simulink model "hopper_3dof_cascade_No_wind - Copy"  (R2025a)
settings: Solver=VariableStepAuto  StartTime=0.0  StopTime=60  MaxStep=.005  RelTol=1e-3
values from neighbouring files (symbols this model uses):
  AVI = size_avionics(IN)    [main.m]
  bp = data(:,1)    [load_lookup.m]
  ENGINE = size_engine(IN)    [main.m]
  IN =     [hopper_sizing_output.mat]    (also in main.m = mission_inputs())
  OUT =     [hopper_sizing_output.mat]    (also in main.m = Outputs(IN, VEH, TANKS, STRUCT))
  TANKS = size_tanks(IN)    [main.m]
undefined symbols (not defined in the file or in its folder): tbl1, tbl2
libraries: slpidlib x5, simulink x4, SignalEditorBlockLib x1, cstblocks x1, dspsrcs4 x1
settings Model: Creator=Espin  LastModifiedBy=Espin
settings DebuggingCC: AlgebraicLoopMsg=none

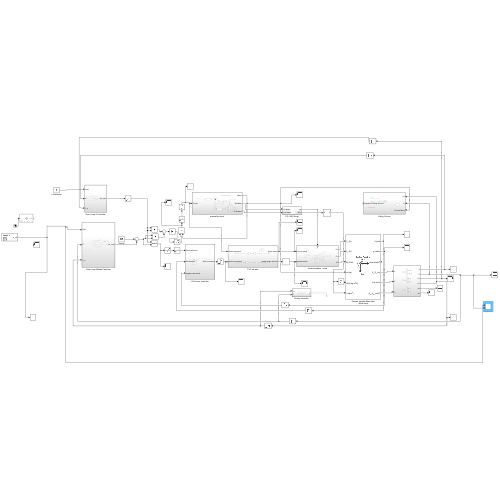
[thumbnail: Simulink's stored preview of the top-level diagram]
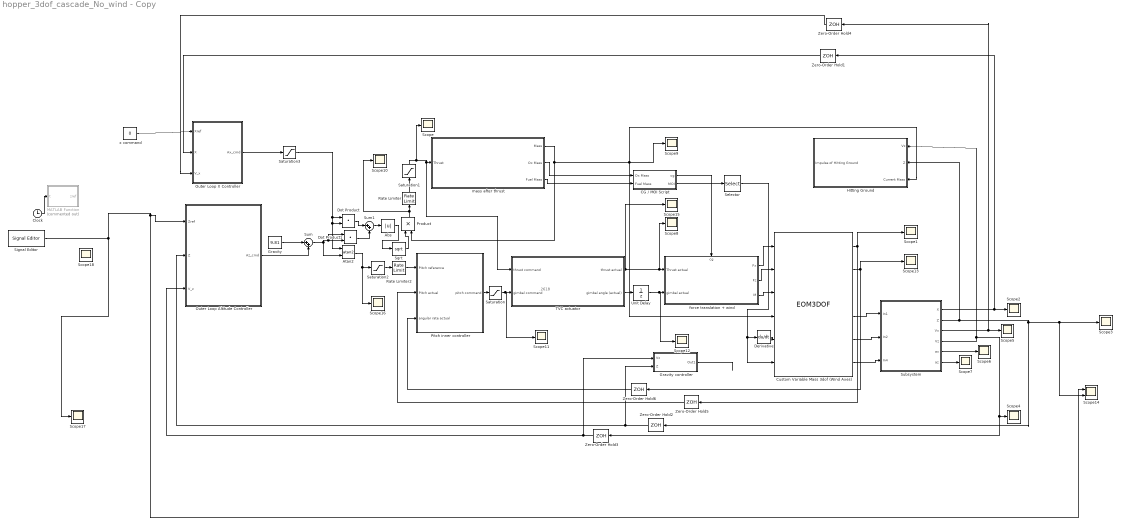
== system hopper_3dof_cascade_No_wind - Copy ==
  note: .2618
  Abs : Abs  SaturateOnIntegerOverflow=off
  Atan2 : Trigonometry  Operator=atan2
  CG / MOI Script : Subsystem
  Clock : Clock
  Custom Variable Mass 3dof (Wind Axes) : EOM3DOF  mtype=Custom Variable  v_ini=0
  Derivative : Derivative
  Dot Product : DotProduct  OutDataTypeStr=Inherit: Inherit via internal rule
  Dot Product1 : DotProduct  OutDataTypeStr=Inherit: Inherit via internal rule
  Gravity : Constant  Value=9.81
  Gravity controller : Subsystem
  Hitting Ground : Subsystem
  MATLAB Function : MATLAB Function  Commented=on  TreatAsAtomicUnit=on
  Outer Loop Altitude Controller : Subsystem
  Outer Loop X Controller : Subsystem
  Pitch inner controller : Subsystem
  Product : Product
  Rate Limiter : RateLimiter  RisingSlewLimit=800  FallingSlewLimit=-800  SampleTimeMode=inherited
  Rate Limiter2 : RateLimiter  RisingSlewLimit=.2618  FallingSlewLimit=-.2618  SampleTimeMode=inherited
  Saturation : Saturate  UpperLimit=.25  LowerLimit=-.25
  Saturation1 : Saturate  UpperLimit=2400  LowerLimit=890  ZeroCross=off
  Saturation2 : Saturate  UpperLimit=.1  LowerLimit=-.1
  Saturation3 : Saturate  UpperLimit=.8  LowerLimit=-.8
  Scope{,1..13,15..18} (18 alike) : Scope
      Scope settings: ActiveDisplayYMinimum=624.4996725299402  ActiveDisplayYMaximum=2705.46842252994  DataLoggingVariableName=ScopeData17
      Scope1 settings: ActiveDisplayYMinimum=-3.9694175819180568  ActiveDisplayYMaximum=3.8842046224775704  DataLoggingVariableName=ScopeData4
      Scope10 settings: ActiveDisplayYMinimum=-1  ActiveDisplayYMaximum=1  DataLoggingVariableName=ScopeData18
      Scope11 settings: ActiveDisplayYMinimum=-0.486354941657661  ActiveDisplayYMaximum=0.24913214764343761  DataLoggingVariableName=ScopeData19
      Scope12 settings: ActiveDisplayYMinimum=-1.2645796500990321  ActiveDisplayYMaximum=0.59395959390663888  DataLoggingVariableName=ScopeData20
      Scope13 settings: ActiveDisplayYMinimum=0.23771889209507596  ActiveDisplayYMaximum=0.35709262601864444  DataLoggingVariableName=ScopeData21
      Scope15 settings: ActiveDisplayYMinimum=931.27769507113021  ActiveDisplayYMaximum=1211.8430429766809  DataLoggingVariableName=ScopeData25
      Scope16 settings: ActiveDisplayYMinimum=-0.10872394180597797  ActiveDisplayYMaximum=0.024612722486554474  DataLoggingVariableName=ScopeData26
      Scope17 settings: ActiveDisplayYMinimum=-6.2499999999999982  ActiveDisplayYMaximum=56.25  DataLoggingVariableName=ScopeData31
      Scope18 settings: ActiveDisplayYMinimum=-6.2499999999999982  ActiveDisplayYMaximum=56.25  DataLoggingVariableName=ScopeData39
      Scope2 settings: ActiveDisplayYMinimum=-3413.3164906748493  ActiveDisplayYMaximum=7586.6291552550156  DataLoggingVariableName=ScopeData6
      Scope3 settings: ActiveDisplayYMinimum=-1202.9630045130734  ActiveDisplayYMaximum=1936.8327091689698  DataLoggingVariableName=ScopeData7
      Scope4 settings: ActiveDisplayYMinimum=-29.297460678782883  ActiveDisplayYMaximum=38.963570912357639
      Scope5 settings: ActiveDisplayYMinimum=-962.2230612403514  ActiveDisplayYMaximum=1558.6587762750428  DataLoggingVariableName=ScopeData9
      Scope6 settings: ActiveDisplayYMinimum=-962.2230612403514  ActiveDisplayYMaximum=1558.6587762750428  DataLoggingVariableName=ScopeData10
      Scope7 settings: ActiveDisplayYMinimum=-962.2230612403514  ActiveDisplayYMaximum=1558.6587762750428  DataLoggingVariableName=ScopeData11
      Scope8 settings: ActiveDisplayYMinimum=931.27769507113021  ActiveDisplayYMaximum=1211.8430429766809  DataLoggingVariableName=ScopeData12
      Scope9 settings: ActiveDisplayYMinimum=94.915833260187526  ActiveDisplayYMaximum=94.915892608014829  DataLoggingVariableName=ScopeData13
  Scope14 : Scope  NumInputPorts=2
      settings: ActiveDisplayYMinimum=-2.6899782864025186  ActiveDisplayYMaximum=3.1359753018738186  DataLoggingVariableName=ScopeData22
  Selector : Selector  NumberOfDimensions=2  InputPortWidth=1  IndexOptions=Index vector (dialog),Index vector (dialog)  Indices=2,2  OutputSizes=1,1
  Signal Editor : SignalEditorBlockLib/Signal Editor  FileName=trajectory2.mat  ActiveScenario=scenario  ActiveSignal=z_ref  IsBus=off  OutputBusObjectStr=Bus: BusObject  SampleTime=0  ZeroCross=off  OutputAfterFinalValue=Setting to zero  Unit=inherit  PreserveSignalName=on  ApplySigPropsToAllScenarios=on  ApplySigPropsToAllSignals=off  SignalPropertySource=Dialog parameters
  Sqrt : Sqrt
  Subsystem : Subsystem
  Sum : Sum  Inputs=|++
  Sum1 : Sum  Inputs=|++
  TVC actuator : Subsystem
  Unit Delay : UnitDelay  SampleTime=-1  HasFrameUpgradeWarning=on
  Zero-Order Hold{1..6} (6 alike) : ZeroOrderHold  SampleTime=-1
  force translation + wind : Subsystem
      settings: PortSchema="{\"entries\":[{\"content\":{\"sides\":[{\"content\":{\"connectorIds\":[\"In1\",\"In2\"]},\"type\":\"ConnectorPlacement.EquallySpacedRectSide\",\"uuid\":\"479fd6fb-19b9-4dfd-bf6b-42f12e82a54f\"},{\"content\":{\"connectorIds\":[\"Out1\",\"Out2\",\"Out3\"],\"side\":\"RIGHT\"},\"type\":\"ConnectorPlacement.EquallySpacedRectSide\",\"uuid\":\"4df03b8d-1b7e-4664-b5ef-d45791de0677\"},{\"content\":{\"connectorIds\":[\"In3\"],\"side\":\"TOP\"},\"type\":\"ConnectorPlacement.EquallySpacedRectSide\",\"uuid\":\"8e173f4c-8dd7-429b-b7ff-7241e32a3938\"}]},\"type\":\"ConnectorPlacement.EquallySpacedConnector\",\"uuid\":\"4fb4042b-69d2-4473-a071-5f8ab2a018ab\"}],\"packageUris\":[\"http://schema.mathworks.com/mf0/Connector/R2020b\"],\"version\":\"1.0\"}"
  mass after thrust : Subsystem
  x command : Constant  Value=0
  wires:
  Custom Variable Mass 3dof (Wind Axes)/6 -> Subsystem/3(In4)
  Custom Variable Mass 3dof (Wind Axes)/5 -> Subsystem/2(In2)
  Custom Variable Mass 3dof (Wind Axes)/4 -> Subsystem/1(In1)
  Atan2/1 -> Scope16/1, Saturation2/1
  Pitch inner controller/1(pitch command) -> Saturation/1
  Saturation/1 -> Scope11/1, TVC actuator/2(gimbal command)
  Gravity/1 -> Sum/1
  mass after thrust/1(Mass) -> Product/2, Hitting Ground/3(Current Mass), Scope9/1, Custom Variable Mass 3dof (Wind Axes)/4
  Rate Limiter/1 -> Saturation1/1
  Product/1 -> Scope10/1, Rate Limiter/1
  Custom Variable Mass 3dof (Wind Axes)/1 -> Scope1/1, Zero-Order Hold5/1
  Custom Variable Mass 3dof (Wind Axes)/2 -> Scope13/1, Zero-Order Hold6/1
  Subsystem/1(X) -> Zero-Order Hold1/1, Scope2/1
  Subsystem/2(Z) -> Hitting Ground/2(Z), Zero-Order Hold2/1, Scope14/2, Scope3/1
  force translation + wind/1(Fx) -> Custom Variable Mass 3dof (Wind Axes)/1
  force translation + wind/3(M) -> Custom Variable Mass 3dof (Wind Axes)/3
  force translation + wind/2(Fz) -> Custom Variable Mass 3dof (Wind Axes)/2
  Subsystem/4(Vz) -> Hitting Ground/1(Vz), Zero-Order Hold3/1, Scope4/1
  Subsystem/3(Vx) -> Zero-Order Hold4/1, Scope5/1
  Subsystem/5(ax) -> Scope6/1
  Subsystem/6(az) -> Scope7/1
  Signal Editor/1 -> Scope14/1, Outer Loop Altitude Controller/1(Zref), Scope17/1
  Outer Loop Altitude Controller/1(Az_cmd) -> Sum/2
  Sqrt/1 -> Product/1
  x command/1 -> Outer Loop X Controller/1(Xref)
  Sum/1 -> Dot Product1/1, Dot Product1/2, Atan2/2
  Dot Product/1 -> Sum1/1
  Sum1/1 -> Abs/1
  Dot Product1/1 -> Sum1/2
  Abs/1 -> Sqrt/1
  Outer Loop X Controller/1(Ax_cmd) -> Saturation3/1
  Saturation1/1 -> Scope/1, TVC actuator/1(thrust command), mass after thrust/1(Thrust)
  Zero-Order Hold1/1 -> Outer Loop X Controller/2(X)
  Zero-Order Hold4/1 -> Outer Loop X Controller/3(V_x)
  Zero-Order Hold3/1 -> Gravity controller/1(Vz), Outer Loop Altitude Controller/3(V_z)
  Zero-Order Hold2/1 -> Gravity controller/2(Z), Outer Loop Altitude Controller/2(Z)
  Zero-Order Hold5/1 -> Pitch inner controller/2(Pitch actual)
  Zero-Order Hold6/1 -> Pitch inner controller/3(angular rate actual)
  TVC actuator/2(gimbal angle (actual)) -> Unit Delay/1
  Unit Delay/1 -> Scope12/1, force translation + wind/2(gimbal actual)
  TVC actuator/1(thrust actual) -> Scope8/1, force translation + wind/1(Thrust actual), Scope15/1
  Saturation2/1 -> Rate Limiter2/1
  Rate Limiter2/1 -> Pitch inner controller/1(Pitch reference)
  Saturation3/1 -> Dot Product/1, Atan2/1, Dot Product/2
  mass after thrust/2(Ox Mass) -> CG / MOI Script/1(Ox Mass)
  mass after thrust/3(Fuel Mass) -> CG / MOI Script/2(Fuel Mass)
  CG / MOI Script/1(cg) -> force translation + wind/3(cg)
  Derivative/1 -> Custom Variable Mass 3dof (Wind Axes)/5
  CG / MOI Script/2(MOI) -> Selector/1
  Selector/1 -> Custom Variable Mass 3dof (Wind Axes)/6, Derivative/1
  Clock/1 -> MATLAB Function/1(t)
  Gravity controller/1(Out1) -> ?

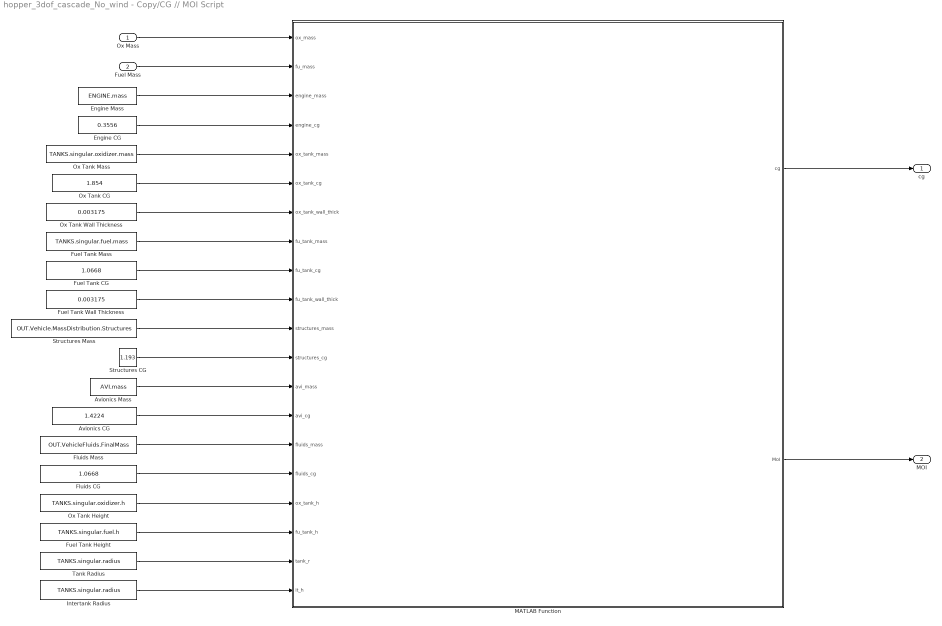
== system hopper_3dof_cascade_No_wind - Copy/CG // MOI Script ==
  Ox Mass : Inport
  Fuel Mass : Inport  Port=2
  Avionics CG : Constant  Value=1.4224
  Avionics Mass : Constant  Value=AVI.mass
  Engine CG : Constant  Value=0.3556
  Engine Mass : Constant  Value=ENGINE.mass
  Fluids CG : Constant  Value=1.0668
  Fluids Mass : Constant  Value=OUT.VehicleFluids.FinalMass
  Fuel Tank CG : Constant  Value=1.0668
  Fuel Tank Height : Constant  Value=TANKS.singular.fuel.h
  Fuel Tank Mass : Constant  Value=TANKS.singular.fuel.mass
  Fuel Tank Wall Thickness : Constant  Value=0.003175
  Intertank Radius : Constant  Value=TANKS.singular.radius
  MATLAB Function : MATLAB Function  TreatAsAtomicUnit=on
  Ox Tank CG : Constant  Value=1.854
  Ox Tank Height : Constant  Value=TANKS.singular.oxidizer.h
  Ox Tank Mass : Constant  Value=TANKS.singular.oxidizer.mass
  Ox Tank Wall Thickness : Constant  Value=0.003175
  Structures CG : Constant  Value=1.193
  Structures Mass : Constant  Value=OUT.Vehicle.MassDistribution.Structures
  Tank Radius : Constant  Value=TANKS.singular.radius
  cg : Outport
  MOI : Outport  Port=2
  wires:
  Ox Mass/1 -> MATLAB Function/1(ox_mass)
  Fuel Mass/1 -> MATLAB Function/2(fu_mass)
  Engine Mass/1 -> MATLAB Function/3(engine_mass)
  Engine CG/1 -> MATLAB Function/4(engine_cg)
  Ox Tank Mass/1 -> MATLAB Function/5(ox_tank_mass)
  Ox Tank CG/1 -> MATLAB Function/6(ox_tank_cg)
  Ox Tank Wall Thickness/1 -> MATLAB Function/7(ox_tank_wall_thick)
  Fuel Tank Mass/1 -> MATLAB Function/8(fu_tank_mass)
  Fuel Tank CG/1 -> MATLAB Function/9(fu_tank_cg)
  Fuel Tank Wall Thickness/1 -> MATLAB Function/10(fu_tank_wall_thick)
  Structures Mass/1 -> MATLAB Function/11(structures_mass)
  Structures CG/1 -> MATLAB Function/12(structures_cg)
  Avionics Mass/1 -> MATLAB Function/13(avi_mass)
  Avionics CG/1 -> MATLAB Function/14(avi_cg)
  Fluids Mass/1 -> MATLAB Function/15(fluids_mass)
  Fluids CG/1 -> MATLAB Function/16(fluids_cg)
  Ox Tank Height/1 -> MATLAB Function/17(ox_tank_h)
  Fuel Tank Height/1 -> MATLAB Function/18(fu_tank_h)
  Tank Radius/1 -> MATLAB Function/19(tank_r)
  Intertank Radius/1 -> MATLAB Function/20(it_h)
  MATLAB Function/2(MoI) -> MOI/1
  MATLAB Function/1(cg) -> cg/1

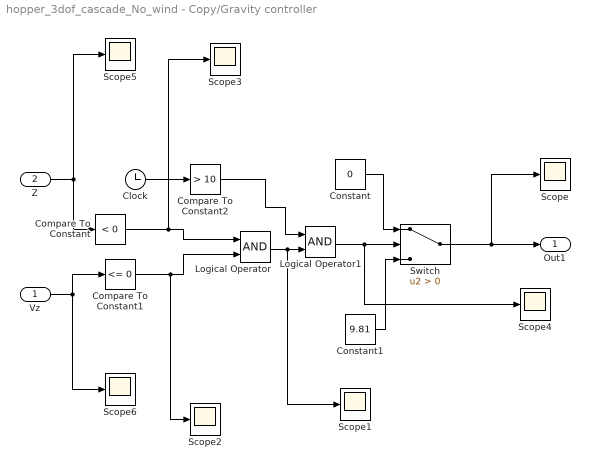
== system hopper_3dof_cascade_No_wind - Copy/Gravity controller ==
  Vz : Inport
  Z : Inport  Port=2
  Clock : Clock
  Compare To Constant : simulink/Logic and Bit Operations/Compare To Constant  relop=<  const=0  OutDataTypeStr=boolean
  Compare To Constant1 : simulink/Logic and Bit Operations/Compare To Constant  relop=<=  const=0  OutDataTypeStr=boolean
  Compare To Constant2 : simulink/Logic and Bit Operations/Compare To Constant  relop=>  const=10  OutDataTypeStr=boolean
  Constant : Constant  Value=0
  Constant1 : Constant  Value=9.81
  Logical Operator : Logic  AllPortsSameDT=off  OutDataTypeStr=boolean
  Logical Operator1 : Logic  AllPortsSameDT=off  OutDataTypeStr=boolean
  Scope{,1..6} (7 alike) : Scope
      Scope settings: ActiveDisplayYMinimum=-0.8627829911971161  ActiveDisplayYMaximum=3.9899046567195673  DataLoggingVariableName=ScopeData32
      Scope1 settings: ActiveDisplayYMinimum=-1  ActiveDisplayYMaximum=1  DataLoggingVariableName=ScopeData33
      Scope2 settings: ActiveDisplayYMinimum=-1  ActiveDisplayYMaximum=1  DataLoggingVariableName=ScopeData34
      Scope3 settings: ActiveDisplayYMinimum=0.16297275299479574  ActiveDisplayYMaximum=1.8744028088981914  DataLoggingVariableName=ScopeData35
      Scope4 settings: ActiveDisplayYMinimum=-1  ActiveDisplayYMaximum=1  DataLoggingVariableName=ScopeData36
      Scope5 settings: ActiveDisplayYMinimum=-1.0594311377245509  ActiveDisplayYMaximum=1.0405688622754492  DataLoggingVariableName=ScopeData37
      Scope6 settings: ActiveDisplayYMinimum=-1.2262499999999998  ActiveDisplayYMaximum=11.03625  DataLoggingVariableName=ScopeData38
  Switch : Switch  Criteria=u2 > Threshold  SaturateOnIntegerOverflow=off  InputSameDT=off
  Out1 : Outport
  wires:
  Vz/1 -> Scope6/1, Compare To Constant1/1
  Z/1 -> Scope5/1, Compare To Constant/1
  Compare To Constant1/1 -> Scope2/1, Logical Operator/2
  Compare To Constant/1 -> Scope3/1, Logical Operator/1
  Clock/1 -> Compare To Constant2/1
  Compare To Constant2/1 -> Logical Operator1/1
  Logical Operator/1 -> Scope1/1, Logical Operator1/2
  Logical Operator1/1 -> Scope4/1, Switch/2
  Constant1/1 -> Switch/3
  Constant/1 -> Switch/1
  Switch/1 -> Scope/1, Out1/1

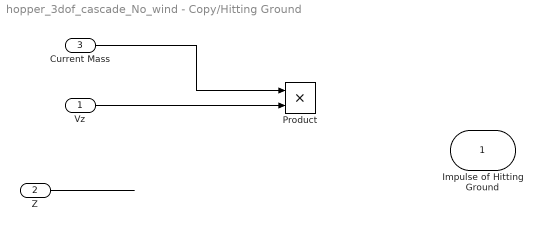
== system hopper_3dof_cascade_No_wind - Copy/Hitting Ground ==
  Vz : Inport
  Z : Inport  Port=2
  Current Mass : Inport  Port=3
  Product : Product
  Impulse of Hitting Ground : Outport
  wires:
  Vz/1 -> Product/2
  Z/1 -> ?
  Current Mass/1 -> Product/1

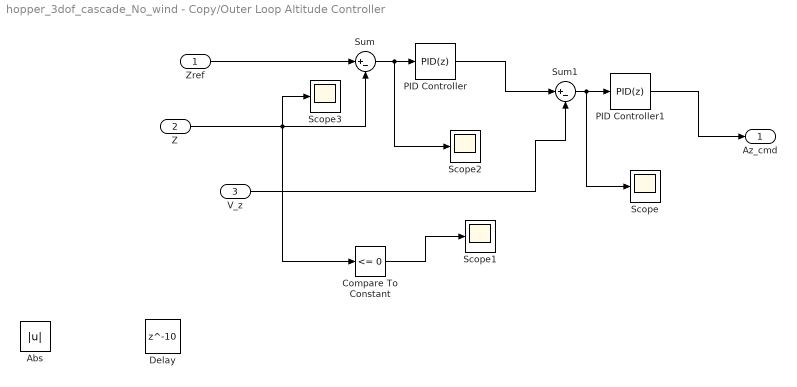
== system hopper_3dof_cascade_No_wind - Copy/Outer Loop Altitude Controller ==
  Zref : Inport
  Z : Inport  Port=2
  V_z : Inport  Port=3
  Abs : Abs  SaturateOnIntegerOverflow=off
  Compare To Constant : simulink/Logic and Bit Operations/Compare To Constant  relop=<=  const=0  OutDataTypeStr=boolean
  Delay : Delay  DelayLength=10  InitialCondition=0
  PID Controller : slpidlib/PID Controller  Controller=PID  Form=Parallel  TimeDomain=Discrete-time  UseExternalTs=off  SampleTime=.02  IntegratorMethod=Forward Euler  FilterMethod=Forward Euler  ControllerParametersSource=internal  P=1  I=0  UseKiTs=off  D=0  UseExternalDerivativeSource=off  N=71.8360137365129  UseFilter=off  TunerSelectOption=Transfer Function Based (PID Tuner App)  InitialConditionSource=internal  InitialConditionForIntegrator=0  InitialConditionForFilter=0  DifferentiatorICPrevScaledInput=0  ExternalReset=none  TrackingMode=off  Kt=1  LimitOutput=off  SatLimitsSource=internal  UpperSaturationLimit=inf  LowerSaturationLimit=-inf  LinearizeAsGain=on  AntiWindupMode=none  Kb=1  LimitIntegrator=off  UpperIntegratorSaturationLimit=inf  LowerIntegratorSaturationLimit=-inf  POutMin=[]  POutMax=[]  IOutMin=[]  IOutMax=[]  DOutMin=[]  DOutMax=[]  NOutMin=[]  NOutMax=[]  SumOutMin=[]  SumOutMax=[]  SaturationOutMin=[]  SaturationOutMax=[]  PParamMin=[]  PParamMax=[]  IParamMin=[]  IParamMax=[]  DParamMin=[]  DParamMax=[]  NParamMin=[]  NParamMax=[]  KbParamMin=[]  KbParamMax=[]  KtParamMin=[]  KtParamMax=[]  KbOutMin=[]  KbOutMax=[]  KtOutMin=[]  KtOutMax=[]  IntegratorOutMin=[]  IntegratorOutMax=[]  FilterOutMin=[]  FilterOutMax=[]  SumI1OutMin=[]  SumI1OutMax=[]  SumI2OutMin=[]  SumI2OutMax=[]  SumI3OutMin=[]  SumI3OutMax=[]  SumI4OutMin=[]  SumI4OutMax=[]  SumDOutMin=[]  SumDOutMax=[]  DifferentiatorOutMin=[]  DifferentiatorOutMax=[]  FilterDiffOutCoefMin=[]  FilterDiffOutCoefMax=[]  ReciprocalOutMin=[]  ReciprocalOutMax=[]  SumDenOutMin=[]  SumDenOutMax=[]  SumNumOutMin=[]  SumNumOutMax=[]  DivideOutMin=[]  DivideOutMax=[]  UdiffTsProdOutMin=[]  UdiffTsProdOutMax=[]  NTsProdOutMin=[]  NTsProdOutMax=[]  UintegralTsProdOutMin=[]  UintegralTsProdOutMax=[]  UngainTsProdOutMin=[]  UngainTsProdOutMax=[]  ClampingZeroOutDataTypeStr=Inherit: Inherit via back propagation  ClampingZeroOutMin=[]  ClampingZeroOutMax=[]  FilterDenConstantOutDataTypeStr=Inherit: Inherit via back propagation  FilterDenConstantOutMin=[]  FilterDenConstantOutMax=[]  PCopyOutDataTypeStr=Inherit: Inherit via back propagation  PCopyOutMin=[]  PCopyOutMax=[]  NCopyOutDataTypeStr=Inherit: Inherit via back propagation  NCopyOutMin=[]  NCopyOutMax=[]  IntegratorContinuousStateAttributes=''  IntegratorStateMustResolveToSignalObject=off  IntegratorRTWStateStorageClass=Auto  FilterContinuousStateAttributes=''  FilterStateMustResolveToSignalObject=off  FilterRTWStateStorageClass=Auto  ParallelPVariant=InternalParameters  IdealPVariant=Disabled  IVariant=InternalParameters  DVariant=InternalParameters  IntegratorVariant=Discrete  SatVariant=Disabled  AWVariant=Passthrough  PCopyVariant=Disabled  TRVariant=Disabled  FdbkBlocksVariant=Forward  IdealPFdbkVariant=Disabled  SatFdbkVariant=Disabled  DerivativeFilterVariant=Differentiator  NVariant=Passthrough  NCopyVariant=Disabled_SignalSpec  FilterICVariant=InternalICsDifferentiator  IntegratorICVariant=InternalICs  ExternalResetVariant=Disabled  TRSumVariant=Passthrough  SumFdbkVariant=Disabled  SumVariant=Sum_PID  TsampFilterVariant=InternalTs  TsampNgainVariant=Passthrough  TsampIntegralVariant=Disabled_SignalSpec  ExternalSaturationOutDataTypeStr=Inherit: Same as second input  DerivativeSourceVariant=ErrorSignal  PreIntVariant=InternalPreInt
  PID Controller1 : slpidlib/PID Controller  Controller=PID  Form=Parallel  TimeDomain=Discrete-time  UseExternalTs=off  SampleTime=.02  IntegratorMethod=Forward Euler  FilterMethod=Forward Euler  ControllerParametersSource=internal  P=-4.85683929346037  I=-2.4299931951401  UseKiTs=off  D=-0.135933719312933  UseExternalDerivativeSource=off  N=71.8360137365129  UseFilter=off  TunerSelectOption=Transfer Function Based (PID Tuner App)  InitialConditionSource=internal  InitialConditionForIntegrator=0  InitialConditionForFilter=0  DifferentiatorICPrevScaledInput=0  ExternalReset=none  TrackingMode=off  Kt=1  LimitOutput=off  SatLimitsSource=internal  UpperSaturationLimit=inf  LowerSaturationLimit=-inf  LinearizeAsGain=on  AntiWindupMode=none  Kb=1  LimitIntegrator=off  UpperIntegratorSaturationLimit=inf  LowerIntegratorSaturationLimit=-inf  POutMin=[]  POutMax=[]  IOutMin=[]  IOutMax=[]  DOutMin=[]  DOutMax=[]  NOutMin=[]  NOutMax=[]  SumOutMin=[]  SumOutMax=[]  SaturationOutMin=[]  SaturationOutMax=[]  PParamMin=[]  PParamMax=[]  IParamMin=[]  IParamMax=[]  DParamMin=[]  DParamMax=[]  NParamMin=[]  NParamMax=[]  KbParamMin=[]  KbParamMax=[]  KtParamMin=[]  KtParamMax=[]  KbOutMin=[]  KbOutMax=[]  KtOutMin=[]  KtOutMax=[]  IntegratorOutMin=[]  IntegratorOutMax=[]  FilterOutMin=[]  FilterOutMax=[]  SumI1OutMin=[]  SumI1OutMax=[]  SumI2OutMin=[]  SumI2OutMax=[]  SumI3OutMin=[]  SumI3OutMax=[]  SumI4OutMin=[]  SumI4OutMax=[]  SumDOutMin=[]  SumDOutMax=[]  DifferentiatorOutMin=[]  DifferentiatorOutMax=[]  FilterDiffOutCoefMin=[]  FilterDiffOutCoefMax=[]  ReciprocalOutMin=[]  ReciprocalOutMax=[]  SumDenOutMin=[]  SumDenOutMax=[]  SumNumOutMin=[]  SumNumOutMax=[]  DivideOutMin=[]  DivideOutMax=[]  UdiffTsProdOutMin=[]  UdiffTsProdOutMax=[]  NTsProdOutMin=[]  NTsProdOutMax=[]  UintegralTsProdOutMin=[]  UintegralTsProdOutMax=[]  UngainTsProdOutMin=[]  UngainTsProdOutMax=[]  ClampingZeroOutDataTypeStr=Inherit: Inherit via back propagation  ClampingZeroOutMin=[]  ClampingZeroOutMax=[]  FilterDenConstantOutDataTypeStr=Inherit: Inherit via back propagation  FilterDenConstantOutMin=[]  FilterDenConstantOutMax=[]  PCopyOutDataTypeStr=Inherit: Inherit via back propagation  PCopyOutMin=[]  PCopyOutMax=[]  NCopyOutDataTypeStr=Inherit: Inherit via back propagation  NCopyOutMin=[]  NCopyOutMax=[]  IntegratorContinuousStateAttributes=''  IntegratorStateMustResolveToSignalObject=off  IntegratorRTWStateStorageClass=Auto  FilterContinuousStateAttributes=''  FilterStateMustResolveToSignalObject=off  FilterRTWStateStorageClass=Auto  ParallelPVariant=InternalParameters  IdealPVariant=Disabled  IVariant=InternalParameters  DVariant=InternalParameters  IntegratorVariant=Discrete  SatVariant=Disabled  AWVariant=Passthrough  PCopyVariant=Disabled  TRVariant=Disabled  FdbkBlocksVariant=Forward  IdealPFdbkVariant=Disabled  SatFdbkVariant=Disabled  DerivativeFilterVariant=Differentiator  NVariant=Passthrough  NCopyVariant=Disabled_SignalSpec  FilterICVariant=InternalICsDifferentiator  IntegratorICVariant=InternalICs  ExternalResetVariant=Disabled  TRSumVariant=Passthrough  SumFdbkVariant=Disabled  SumVariant=Sum_PID  TsampFilterVariant=InternalTs  TsampNgainVariant=Passthrough  TsampIntegralVariant=Disabled_SignalSpec  ExternalSaturationOutDataTypeStr=Inherit: Same as second input  DerivativeSourceVariant=ErrorSignal  PreIntVariant=InternalPreInt
  Scope{,1..3} (4 alike) : Scope
      Scope settings: ActiveDisplayYMinimum=-3022.4394216854653  ActiveDisplayYMaximum=1190.9746216235139  DataLoggingVariableName=ScopeData27
      Scope1 settings: ActiveDisplayYMinimum=-100.23822529551113  ActiveDisplayYMaximum=60.856281885106874  DataLoggingVariableName=ScopeData28
      Scope2 settings: ActiveDisplayYMinimum=-1450.1308335174933  ActiveDisplayYMaximum=480.08268664272219  DataLoggingVariableName=ScopeData29
      Scope3 settings: ActiveDisplayYMinimum=-2628.2294879970932  ActiveDisplayYMaximum=1011.4759807937319  DataLoggingVariableName=ScopeData30
  Sum : Sum  Inputs=|+-
  Sum1 : Sum  Inputs=|+-
  Az_cmd : Outport
  wires:
  Zref/1 -> Sum/1
  PID Controller1/1 -> Az_cmd/1
  Sum/1 -> Scope2/1, PID Controller/1
  V_z/1 -> Sum1/2
  Sum1/1 -> Scope/1, PID Controller1/1
  Compare To Constant/1 -> Scope1/1
  Z/1 -> Scope3/1, Compare To Constant/1, Sum/2
  PID Controller/1 -> Sum1/1

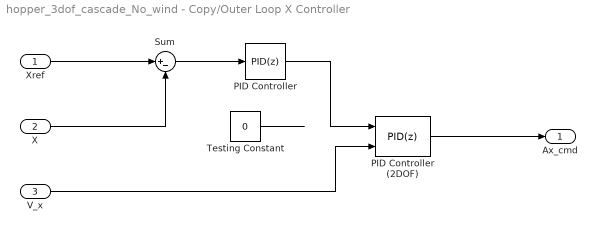
== system hopper_3dof_cascade_No_wind - Copy/Outer Loop X Controller ==
  Xref : Inport
  X : Inport  Port=2
  V_x : Inport  Port=3
  PID Controller : slpidlib/PID Controller  Controller=PID  Form=Parallel  TimeDomain=Discrete-time  UseExternalTs=off  SampleTime=0.02  IntegratorMethod=Forward Euler  FilterMethod=Forward Euler  ControllerParametersSource=internal  P=.1  I=0  UseKiTs=off  D=0  UseExternalDerivativeSource=off  N=3.72873135160004  UseFilter=on  TunerSelectOption=Transfer Function Based (PID Tuner App)  InitialConditionSource=internal  InitialConditionForIntegrator=0  InitialConditionForFilter=0  DifferentiatorICPrevScaledInput=0  ExternalReset=none  TrackingMode=off  Kt=1  LimitOutput=off  SatLimitsSource=internal  UpperSaturationLimit=inf  LowerSaturationLimit=-inf  LinearizeAsGain=on  AntiWindupMode=none  Kb=1  LimitIntegrator=off  UpperIntegratorSaturationLimit=inf  LowerIntegratorSaturationLimit=-inf  POutMin=[]  POutMax=[]  IOutMin=[]  IOutMax=[]  DOutMin=[]  DOutMax=[]  NOutMin=[]  NOutMax=[]  SumOutMin=[]  SumOutMax=[]  SaturationOutMin=[]  SaturationOutMax=[]  PParamMin=[]  PParamMax=[]  IParamMin=[]  IParamMax=[]  DParamMin=[]  DParamMax=[]  NParamMin=[]  NParamMax=[]  KbParamMin=[]  KbParamMax=[]  KtParamMin=[]  KtParamMax=[]  KbOutMin=[]  KbOutMax=[]  KtOutMin=[]  KtOutMax=[]  IntegratorOutMin=[]  IntegratorOutMax=[]  FilterOutMin=[]  FilterOutMax=[]  SumI1OutMin=[]  SumI1OutMax=[]  SumI2OutMin=[]  SumI2OutMax=[]  SumI3OutMin=[]  SumI3OutMax=[]  SumI4OutMin=[]  SumI4OutMax=[]  SumDOutMin=[]  SumDOutMax=[]  DifferentiatorOutMin=[]  DifferentiatorOutMax=[]  FilterDiffOutCoefMin=[]  FilterDiffOutCoefMax=[]  ReciprocalOutMin=[]  ReciprocalOutMax=[]  SumDenOutMin=[]  SumDenOutMax=[]  SumNumOutMin=[]  SumNumOutMax=[]  DivideOutMin=[]  DivideOutMax=[]  UdiffTsProdOutMin=[]  UdiffTsProdOutMax=[]  NTsProdOutMin=[]  NTsProdOutMax=[]  UintegralTsProdOutMin=[]  UintegralTsProdOutMax=[]  UngainTsProdOutMin=[]  UngainTsProdOutMax=[]  ClampingZeroOutDataTypeStr=Inherit: Inherit via back propagation  ClampingZeroOutMin=[]  ClampingZeroOutMax=[]  FilterDenConstantOutDataTypeStr=Inherit: Inherit via back propagation  FilterDenConstantOutMin=[]  FilterDenConstantOutMax=[]  PCopyOutDataTypeStr=Inherit: Inherit via back propagation  PCopyOutMin=[]  PCopyOutMax=[]  NCopyOutDataTypeStr=Inherit: Inherit via back propagation  NCopyOutMin=[]  NCopyOutMax=[]  IntegratorContinuousStateAttributes=''  IntegratorStateMustResolveToSignalObject=off  IntegratorRTWStateStorageClass=Auto  FilterContinuousStateAttributes=''  FilterStateMustResolveToSignalObject=off  FilterRTWStateStorageClass=Auto  ParallelPVariant=InternalParameters  IdealPVariant=Disabled  IVariant=InternalParameters  DVariant=InternalParameters  IntegratorVariant=Discrete  SatVariant=Disabled  AWVariant=Passthrough  PCopyVariant=Disabled  TRVariant=Disabled  FdbkBlocksVariant=Forward  IdealPFdbkVariant=Disabled  SatFdbkVariant=Disabled  DerivativeFilterVariant=ForwardEulerFilter  NVariant=InternalParameters  NCopyVariant=Disabled  FilterICVariant=InternalICsFilter  IntegratorICVariant=InternalICs  ExternalResetVariant=Disabled  TRSumVariant=Passthrough  SumFdbkVariant=Disabled  SumVariant=Sum_PID  TsampFilterVariant=InternalTs  TsampNgainVariant=Passthrough  TsampIntegralVariant=Disabled_SignalSpec  ExternalSaturationOutDataTypeStr=Inherit: Same as second input  DerivativeSourceVariant=ErrorSignal  PreIntVariant=InternalPreInt
  PID Controller (2DOF) : slpidlib/PID Controller (2DOF)  Controller=PID  Form=Parallel  TimeDomain=Discrete-time  UseExternalTs=off  SampleTime=.02  IntegratorMethod=Forward Euler  FilterMethod=Forward Euler  ControllerParametersSource=internal  P=.1  I=0  UseKiTs=off  D=0  UseExternalDerivativeSource=off  N=2.4544899458169  UseFilter=on  b=0.839590287267977  c=0.924906068412836  TunerSelectOption=Transfer Function Based (PID Tuner App)  InitialConditionSource=internal  InitialConditionForIntegrator=0  InitialConditionForFilter=0  DifferentiatorICPrevScaledInput=0  ExternalReset=none  TrackingMode=off  Kt=1  LimitOutput=off  SatLimitsSource=internal  UpperSaturationLimit=inf  LowerSaturationLimit=-inf  LinearizeAsGain=on  AntiWindupMode=none  Kb=1  LimitIntegrator=off  UpperIntegratorSaturationLimit=inf  LowerIntegratorSaturationLimit=-inf  POutMin=[]  POutMax=[]  IOutMin=[]  IOutMax=[]  DOutMin=[]  DOutMax=[]  NOutMin=[]  NOutMax=[]  bOutMin=[]  bOutMax=[]  cOutMin=[]  cOutMax=[]  SumOutMin=[]  SumOutMax=[]  SaturationOutMin=[]  SaturationOutMax=[]  PParamMin=[]  PParamMax=[]  IParamMin=[]  IParamMax=[]  DParamMin=[]  DParamMax=[]  NParamMin=[]  NParamMax=[]  bParamMin=[]  bParamMax=[]  cParamMin=[]  cParamMax=[]  KbParamMin=[]  KbParamMax=[]  KtParamMin=[]  KtParamMax=[]  KbOutMin=[]  KbOutMax=[]  KtOutMin=[]  KtOutMax=[]  IntegratorOutMin=[]  IntegratorOutMax=[]  FilterOutMin=[]  FilterOutMax=[]  SumI1OutMin=[]  SumI1OutMax=[]  SumI2OutMin=[]  SumI2OutMax=[]  SumI3OutMin=[]  SumI3OutMax=[]  SumI4OutMin=[]  SumI4OutMax=[]  SumDOutMin=[]  SumDOutMax=[]  Sum1OutMin=[]  Sum1OutMax=[]  Sum2OutMin=[]  Sum2OutMax=[]  Sum3OutMin=[]  Sum3OutMax=[]  DifferentiatorOutMin=[]  DifferentiatorOutMax=[]  FilterDiffOutCoefMin=[]  FilterDiffOutCoefMax=[]  ReciprocalOutMin=[]  ReciprocalOutMax=[]  SumDenOutMin=[]  SumDenOutMax=[]  SumNumOutMin=[]  SumNumOutMax=[]  DivideOutMin=[]  DivideOutMax=[]  UdiffTsProdOutMin=[]  UdiffTsProdOutMax=[]  NTsProdOutMin=[]  NTsProdOutMax=[]  UintegralTsProdOutMin=[]  UintegralTsProdOutMax=[]  UngainTsProdOutMin=[]  UngainTsProdOutMax=[]  ClampingZeroOutDataTypeStr=Inherit: Inherit via back propagation  ClampingZeroOutMin=[]  ClampingZeroOutMax=[]  FilterDenConstantOutDataTypeStr=Inherit: Inherit via back propagation  FilterDenConstantOutMin=[]  FilterDenConstantOutMax=[]  PCopyOutDataTypeStr=Inherit: Inherit via back propagation  PCopyOutMin=[]  PCopyOutMax=[]  NCopyOutDataTypeStr=Inherit: Inherit via back propagation  NCopyOutMin=[]  NCopyOutMax=[]  IntegratorContinuousStateAttributes=''  IntegratorStateMustResolveToSignalObject=off  IntegratorRTWStateStorageClass=Auto  FilterContinuousStateAttributes=''  FilterStateMustResolveToSignalObject=off  FilterRTWStateStorageClass=Auto  ParallelPVariant=InternalParameters  IdealPVariant=Disabled  IVariant=InternalParameters  DVariant=InternalParameters  bVariant=InternalParameters  cVariant=InternalParameters  IntegratorVariant=Discrete  SatVariant=Disabled  AWVariant=Passthrough  PCopyVariant=Disabled  TRVariant=Disabled  FdbkBlocksVariant=Forward  IdealPFdbkVariant=Disabled  SatFdbkVariant=Disabled  DerivativeFilterVariant=ForwardEulerFilter  NVariant=InternalParameters  NCopyVariant=Disabled  FilterICVariant=InternalICsFilter  IntegratorICVariant=InternalICs  ExternalResetVariant=Disabled  TRSumVariant=Passthrough  SumFdbkVariant=Disabled  SumVariant=Sum_PID  TsampFilterVariant=InternalTs  TsampNgainVariant=Passthrough  TsampIntegralVariant=Disabled_SignalSpec  ExternalSaturationOutDataTypeStr=Inherit: Same as second input  DerivativeSourceVariant=ErrorSignal  PreIntVariant=InternalPreInt
  Sum : Sum  Inputs=|+-
  Testing Constant : Constant  Value=0
  Ax_cmd : Outport
  wires:
  Xref/1 -> Sum/1
  PID Controller (2DOF)/1 -> Ax_cmd/1
  Sum/1 -> PID Controller/1
  X/1 -> Sum/2
  PID Controller/1 -> PID Controller (2DOF)/1
  V_x/1 -> PID Controller (2DOF)/2
  Testing Constant/1 -> ?

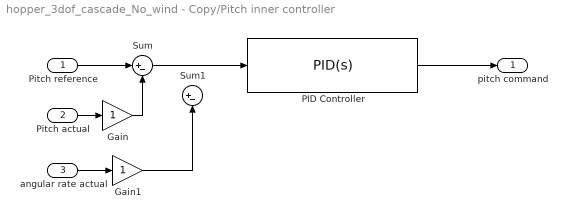
== system hopper_3dof_cascade_No_wind - Copy/Pitch inner controller ==
  Pitch reference : Inport
  Pitch actual : Inport  Port=2
  angular rate actual : Inport  Port=3
  Gain : Gain
  Gain1 : Gain
  PID Controller : slpidlib/PID Controller  Controller=PID  Form=Parallel  TimeDomain=Continuous-time  UseExternalTs=off  SampleTime=.02  IntegratorMethod=Forward Euler  FilterMethod=Forward Euler  ControllerParametersSource=internal  P=-0.000198457505729063  I=-9.23294323293437e-07  UseKiTs=off  D=-0.0270681110655677  UseExternalDerivativeSource=off  N=31.9117250951012  UseFilter=on  TunerSelectOption=Transfer Function Based (PID Tuner App)  InitialConditionSource=internal  InitialConditionForIntegrator=0  InitialConditionForFilter=0  DifferentiatorICPrevScaledInput=0  ExternalReset=none  TrackingMode=off  Kt=1  LimitOutput=off  SatLimitsSource=internal  UpperSaturationLimit=inf  LowerSaturationLimit=-inf  LinearizeAsGain=on  AntiWindupMode=none  Kb=1  LimitIntegrator=off  UpperIntegratorSaturationLimit=inf  LowerIntegratorSaturationLimit=-inf  POutMin=[]  POutMax=[]  IOutMin=[]  IOutMax=[]  DOutMin=[]  DOutMax=[]  NOutMin=[]  NOutMax=[]  SumOutMin=[]  SumOutMax=[]  SaturationOutMin=[]  SaturationOutMax=[]  PParamMin=[]  PParamMax=[]  IParamMin=[]  IParamMax=[]  DParamMin=[]  DParamMax=[]  NParamMin=[]  NParamMax=[]  KbParamMin=[]  KbParamMax=[]  KtParamMin=[]  KtParamMax=[]  KbOutMin=[]  KbOutMax=[]  KtOutMin=[]  KtOutMax=[]  IntegratorOutMin=[]  IntegratorOutMax=[]  FilterOutMin=[]  FilterOutMax=[]  SumI1OutMin=[]  SumI1OutMax=[]  SumI2OutMin=[]  SumI2OutMax=[]  SumI3OutMin=[]  SumI3OutMax=[]  SumI4OutMin=[]  SumI4OutMax=[]  SumDOutMin=[]  SumDOutMax=[]  DifferentiatorOutMin=[]  DifferentiatorOutMax=[]  FilterDiffOutCoefMin=[]  FilterDiffOutCoefMax=[]  ReciprocalOutMin=[]  ReciprocalOutMax=[]  SumDenOutMin=[]  SumDenOutMax=[]  SumNumOutMin=[]  SumNumOutMax=[]  DivideOutMin=[]  DivideOutMax=[]  UdiffTsProdOutMin=[]  UdiffTsProdOutMax=[]  NTsProdOutMin=[]  NTsProdOutMax=[]  UintegralTsProdOutMin=[]  UintegralTsProdOutMax=[]  UngainTsProdOutMin=[]  UngainTsProdOutMax=[]  ClampingZeroOutDataTypeStr=Inherit: Inherit via back propagation  ClampingZeroOutMin=[]  ClampingZeroOutMax=[]  FilterDenConstantOutDataTypeStr=Inherit: Inherit via back propagation  FilterDenConstantOutMin=[]  FilterDenConstantOutMax=[]  PCopyOutDataTypeStr=Inherit: Inherit via back propagation  PCopyOutMin=[]  PCopyOutMax=[]  NCopyOutDataTypeStr=Inherit: Inherit via back propagation  NCopyOutMin=[]  NCopyOutMax=[]  IntegratorContinuousStateAttributes=''  IntegratorStateMustResolveToSignalObject=off  IntegratorRTWStateStorageClass=Auto  FilterContinuousStateAttributes=''  FilterStateMustResolveToSignalObject=off  FilterRTWStateStorageClass=Auto  ParallelPVariant=InternalParameters  IdealPVariant=Disabled  IVariant=InternalParameters  DVariant=InternalParameters  IntegratorVariant=Continuous  SatVariant=Disabled  AWVariant=Passthrough  PCopyVariant=Disabled  TRVariant=Disabled  FdbkBlocksVariant=Forward  IdealPFdbkVariant=Disabled  SatFdbkVariant=Disabled  DerivativeFilterVariant=ContFilter  NVariant=InternalParameters  NCopyVariant=Disabled  FilterICVariant=InternalICsFilter  IntegratorICVariant=InternalICs  ExternalResetVariant=Disabled  TRSumVariant=Passthrough  SumFdbkVariant=Disabled  SumVariant=Sum_PID  TsampFilterVariant=InternalTs  TsampNgainVariant=Passthrough  TsampIntegralVariant=Disabled_SignalSpec  ExternalSaturationOutDataTypeStr=Inherit: Same as second input  DerivativeSourceVariant=ErrorSignal  PreIntVariant=InternalPreInt
  Sum : Sum  Inputs=|+-
  Sum1 : Sum  Inputs=|+-
  pitch command : Outport
  wires:
  Pitch reference/1 -> Sum/1
  Pitch actual/1 -> Gain/1
  Gain/1 -> Sum/2
  Sum/1 -> PID Controller/1
  PID Controller/1 -> pitch command/1
  angular rate actual/1 -> Gain1/1
  Gain1/1 -> Sum1/2

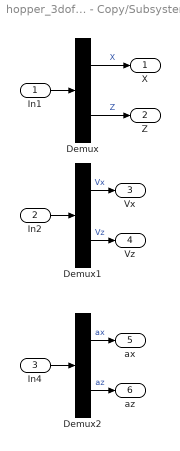
== system hopper_3dof_cascade_No_wind - Copy/Subsystem ==
  In1 : Inport
  In2 : Inport  Port=2
  In4 : Inport  Port=3
  Demux : Demux  Outputs=2
  Demux1 : Demux  Outputs=2
  Demux2 : Demux  Outputs=2
  X : Outport
  Z : Outport  Port=2
  Vx : Outport  Port=3
  Vz : Outport  Port=4
  ax : Outport  Port=5
  az : Outport  Port=6
  wires:
  Demux1/2 -> Vz/1  "Vz"
  In2/1 -> Demux1/1
  Demux1/1 -> Vx/1  "Vx"
  In1/1 -> Demux/1
  Demux/2 -> Z/1  "Z"
  Demux/1 -> X/1  "X"
  Demux2/1 -> ax/1  "ax"
  Demux2/2 -> az/1  "az"
  In4/1 -> Demux2/1

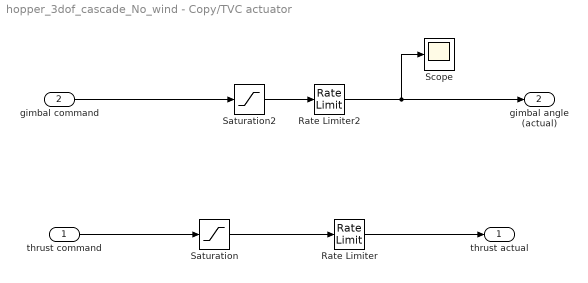
== system hopper_3dof_cascade_No_wind - Copy/TVC actuator ==
  thrust command : Inport
  gimbal command : Inport  Port=2
  Rate Limiter : RateLimiter  RisingSlewLimit=800  FallingSlewLimit=-800  SampleTimeMode=inherited
  Rate Limiter2 : RateLimiter  RisingSlewLimit=.2618  FallingSlewLimit=-.2618  SampleTimeMode=inherited
  Saturation : Saturate  UpperLimit=2400  LowerLimit=890
  Saturation2 : Saturate  UpperLimit=.2618  LowerLimit=-.2618
  Scope : Scope
      settings: ActiveDisplayYMinimum=-0.068803982542027686  ActiveDisplayYMaximum=0.0076448869491141849
  thrust actual : Outport
  gimbal angle (actual) : Outport  Port=2
  wires:
  gimbal command/1 -> Saturation2/1
  Saturation2/1 -> Rate Limiter2/1
  Rate Limiter2/1 -> gimbal angle (actual)/1, Scope/1
  Saturation/1 -> Rate Limiter/1
  thrust command/1 -> Saturation/1
  Rate Limiter/1 -> thrust actual/1

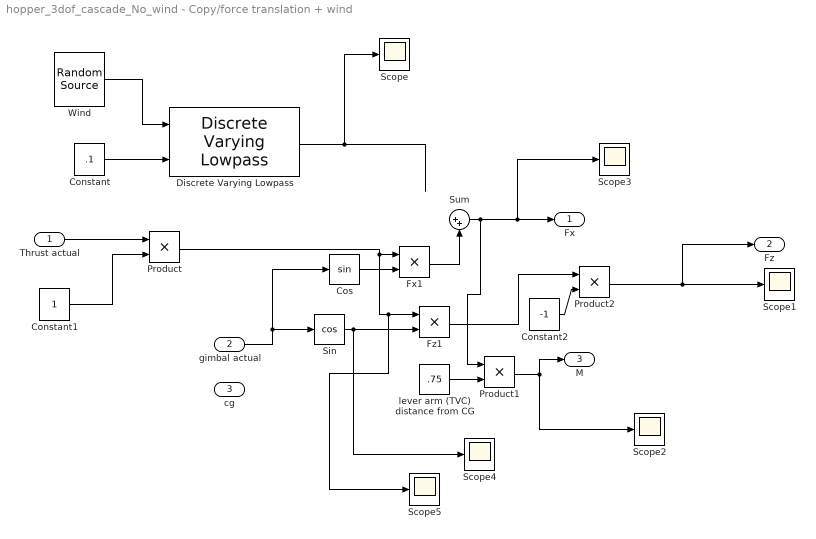
== system hopper_3dof_cascade_No_wind - Copy/force translation + wind ==
  Thrust actual : Inport
  gimbal actual : Inport  Port=2
  cg : Inport  Port=3
  Constant : Constant  Value=.1
  Constant1 : Constant
  Constant2 : Constant  Value=-1
  Cos : Trigonometry
  Discrete Varying Lowpass : cstblocks/Linear Parameter Varying/Discrete Varying Lowpass  N=2  w0=0  Ts=1
  Fx1 : Product
  Fz1 : Product
  Product : Product
  Product1 : Product
  Product2 : Product
  Scope{,1..5} (6 alike) : Scope
      Scope settings: ActiveDisplayYMinimum=-6.7883188179439307  ActiveDisplayYMaximum=61.442213901415776  DataLoggingVariableName=ScopeData8
      Scope1 settings: ActiveDisplayYMinimum=-1  ActiveDisplayYMaximum=1  DataLoggingVariableName=ScopeData14
      Scope2 settings: ActiveDisplayYMinimum=-1  ActiveDisplayYMaximum=1  DataLoggingVariableName=ScopeData15
      Scope3 settings: ActiveDisplayYMinimum=-1  ActiveDisplayYMaximum=1  DataLoggingVariableName=ScopeData16
      Scope4 settings: ActiveDisplayYMinimum=0.96664233806935684  ActiveDisplayYMaximum=0.99127561534918784  DataLoggingVariableName=ScopeData23
      Scope5 settings: ActiveDisplayYMinimum=837.04346660798183  ActiveDisplayYMaximum=1638.9745482042581  DataLoggingVariableName=ScopeData24
  Sin : Trigonometry  Operator=cos
  Sum : Sum  Inputs=|++
  Wind : dspsrcs4/Random Source  SrcType=Gaussian  MinVal=0  MaxVal=1  MeanVal=50  VarVal=1000  RepMode=Specify seed  rawSeed=1  IsInherit=off  SampTime=0.2  SampFrame=1  OutComplex=Real  DataType=double  SimulateUsing=Interpreted execution
  lever arm (TVC) distance from CG : Constant  Value=.75
  Fx : Outport
  Fz : Outport  Port=2
  M : Outport  Port=3
  wires:
  Constant/1 -> Discrete Varying Lowpass/2
  Discrete Varying Lowpass/1 -> Scope/1
  Wind/1 -> Discrete Varying Lowpass/1
  Sum/1 -> Product1/1, Scope3/1, Fx/1
  gimbal actual/1 -> Cos/1, Sin/1
  Product1/1 -> Scope2/1, M/1
  Fx1/1 -> Sum/2
  Sin/1 -> Scope4/1, Fz1/2
  Cos/1 -> Fx1/2
  lever arm (TVC) distance from CG/1 -> Product1/2
  Product/1 -> Scope5/1, Fz1/1, Fx1/1
  Thrust actual/1 -> Product/1
  Constant1/1 -> Product/2
  Fz1/1 -> Product2/1
  Constant2/1 -> Product2/2
  Product2/1 -> Fz/1, Scope1/1

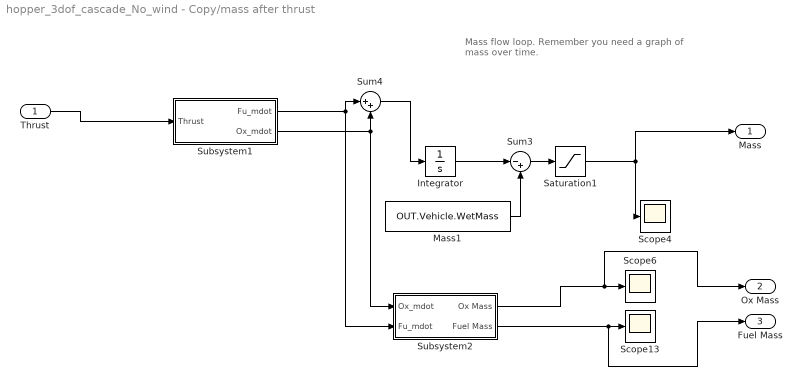
== system hopper_3dof_cascade_No_wind - Copy/mass after thrust ==
  note: Mass flow loop. Remember you need a graph of mass over time.
  Thrust : Inport
  Integrator : Integrator
  Mass1 : Constant  Value=OUT.Vehicle.WetMass
  Saturation1 : Saturate  UpperLimit=OUT.Vehicle.WetMass  LowerLimit=OUT.Vehicle.DryMass
  Scope13 : Scope
      settings: ActiveDisplayYMinimum=-1.1249999999999998  ActiveDisplayYMaximum=10.125  DataLoggingVariableName=ScopeData2
  Scope4 : Scope
      settings: ActiveDisplayYMinimum=87.779536141867183  ActiveDisplayYMaximum=112.03927836942441  DataLoggingVariableName=ScopeData3
  Scope6 : Scope
      settings: ActiveDisplayYMinimum=-1  ActiveDisplayYMaximum=1  DataLoggingVariableName=ScopeData5
  Subsystem1 : Subsystem
  Subsystem2 : Subsystem
  Sum3 : Sum  Inputs=|-+
  Sum4 : Sum  Inputs=|++
  Mass : Outport
  Ox Mass : Outport  Port=2
  Fuel Mass : Outport  Port=3
  wires:
  Thrust/1 -> Subsystem1/1(Thrust)
  Saturation1/1 -> Mass/1, Scope4/1
  Subsystem1/2(Ox_mdot) -> Subsystem2/1(Ox_mdot), Sum4/2
  Mass1/1 -> Sum3/2
  Integrator/1 -> Sum3/1
  Subsystem1/1(Fu_mdot) -> Sum4/1, Subsystem2/2(Fu_mdot)
  Sum3/1 -> Saturation1/1
  Sum4/1 -> Integrator/1
  Subsystem2/2(Fuel Mass) -> Fuel Mass/1, Scope13/1
  Subsystem2/1(Ox Mass) -> Ox Mass/1, Scope6/1

== system hopper_3dof_cascade_No_wind - Copy/mass after thrust/Subsystem1 ==
  Thrust : Inport
  Fuel mdot : Lookup_n-D  NumberOfTableDimensions=1  BreakpointsForDimension1=bp  Table=tbl2  InternalRulePriority=Speed  RndMeth=Simplest
  Ox mdot : Lookup_n-D  NumberOfTableDimensions=1  BreakpointsForDimension1=bp  Table=tbl1  InternalRulePriority=Speed  RndMeth=Simplest
  Fu_mdot : Outport
  Ox_mdot : Outport  Port=2
  wires:
  Thrust/1 -> Ox mdot/1, Fuel mdot/1
  Fuel mdot/1 -> Fu_mdot/1
  Ox mdot/1 -> Ox_mdot/1

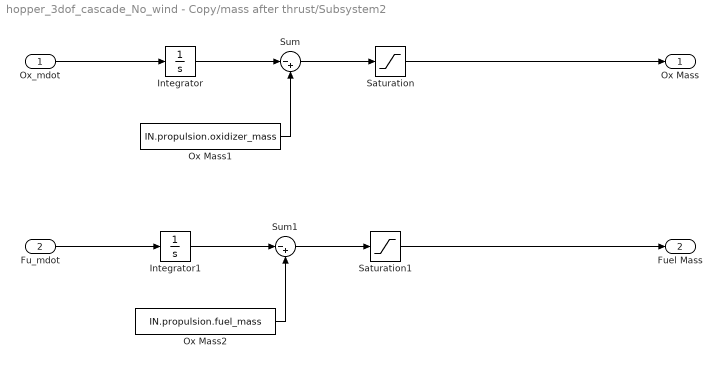
== system hopper_3dof_cascade_No_wind - Copy/mass after thrust/Subsystem2 ==
  Ox_mdot : Inport
  Fu_mdot : Inport  Port=2
  Integrator : Integrator
  Integrator1 : Integrator
  Ox Mass1 : Constant  Value=IN.propulsion.oxidizer_mass
  Ox Mass2 : Constant  Value=IN.propulsion.fuel_mass
  Saturation : Saturate  UpperLimit=IN.propulsion.oxidizer_mass  LowerLimit=0
  Saturation1 : Saturate  UpperLimit=IN.propulsion.fuel_mass  LowerLimit=0
  Sum : Sum  Inputs=|-+
  Sum1 : Sum  Inputs=|-+
  Ox Mass : Outport
  Fuel Mass : Outport  Port=2
  wires:
  Ox_mdot/1 -> Integrator/1
  Integrator/1 -> Sum/1
  Ox Mass1/1 -> Sum/2
  Sum/1 -> Saturation/1
  Saturation/1 -> Ox Mass/1
  Sum1/1 -> Saturation1/1
  Saturation1/1 -> Fuel Mass/1
  Fu_mdot/1 -> Integrator1/1
  Ox Mass2/1 -> Sum1/2
  Integrator1/1 -> Sum1/1

== matlab function hopper_3dof_cascade_No_wind - Copy/MATLAB Function ==
  data: t input; zref output
function zref = z_ref(t)
% Smooth realistic altitude trajectory

zf = 50;        % final altitude (m)
Tup = 14;       % ascent time (s)
Thover = 5;     % hover time (s)
Tdown = 20;     % descent time (s)

% Minimum-jerk profile
mjerk = @(s) (10*s.^3 - 15*s.^4 + 6*s.^5);

if t < 0
    zref = 0;

elseif t < Tup
    s = t / Tup;
    zref = zf * mjerk(s);

elseif t < Tup + Thover
    zref = zf;

elseif t < Tup + Thover + Tdown
    s = (t - (Tup + Thover)) / Tdown;
    zref = zf * (1 - mjerk(s));

else
    zref = 0;
end

== matlab function hopper_3dof_cascade_No_wind - Copy/CG // MOI Script/MATLAB Function ==
  data: ox_mass input; cg output; fu_mass input; engine_mass input; engine_cg input; ox_tank_mass input; ox_tank_cg input; ox_tank_wall_thick input; fu_tank_mass input; fu_tank_cg input; fu_tank_wall_thick input; structures_mass input; structures_cg input; avi_mass input; avi_cg input; fluids_mass input; fluids_cg input; ox_tank_h input; fu_tank_h input; tank_r input; it_h input; MoI output
function [cg, MoI] = cg_sim(ox_mass, fu_mass, engine_mass, engine_cg, ox_tank_mass, ox_tank_cg, ox_tank_wall_thick, fu_tank_mass, fu_tank_cg, fu_tank_wall_thick, structures_mass, structures_cg, avi_mass, avi_cg, fluids_mass, fluids_cg, ox_tank_h, fu_tank_h, tank_r, it_h)
%CG_SIM Calculates the Center of Gravity and Moment of Inertia Matrix
%   Inputs are masses (kg), CG positions (m), and dimensions (m).

    %% 1. Constants and Unit Conversions
    ox_density = 1141;   % kg/m^3
    fu_density = 800;    % kg/m^3
    al_density = 2700;   % kg/m^3 (Density of Al6061)
    
    % Engine dimensions: 4 inch radius, 1 ft length
    eng_r = 4 * 0.0254;  % inches to meters
    eng_h = 1 * 0.3048;  % ft to meters

    %% 2. End Cap Geometry & Mass (NEW)
    % Modeled as solid cylinders attached to the ends of the tank shells.
    % Height of cap = wall thickness of the respective tank.
    
    % --- Oxidizer Tank Caps ---
    h_ox_cap = ox_tank_wall_thick;
    vol_ox_cap = pi * tank_r^2 * h_ox_cap;
    m_ox_cap   = al_density * vol_ox_cap; % Mass of ONE cap
    
    % Positions (Top and Bottom of the hollow shell)
    % Z = Tank_CG +/- (Tank_H/2 + Cap_H/2)
    z_ox_cap_bot = ox_tank_cg - (ox_tank_h / 2) - (h_ox_cap / 2);
    z_ox_cap_top = ox_tank_cg + (ox_tank_h / 2) + (h_ox_cap / 2);

    % --- Fuel Tank Caps ---
    h_fu_cap = fu_tank_wall_thick;
    vol_fu_cap = pi * tank_r^2 * h_fu_cap;
    m_fu_cap   = al_density * vol_fu_cap; % Mass of ONE cap
    
    % Positions
    z_fu_cap_bot = fu_tank_cg - (fu_tank_h / 2) - (h_fu_cap / 2);
    z_fu_cap_top = fu_tank_cg + (fu_tank_h / 2) + (h_fu_cap / 2);

    %% 3. Fluid Geometry Calculations
    % Fuel Fluid
    if fu_mass > 0
        h_fu_fluid = (fu_mass / fu_density) / (pi * tank_r^2);
        % Fluid sits at the bottom of the tank shell
        z_fu_fluid = (fu_tank_cg - fu_tank_h/2) + (h_fu_fluid / 2);
    else
        h_fu_fluid = 0; z_fu_fluid = 0;
    end

    % Oxidizer Fluid
    if ox_mass > 0
        h_ox_fluid = (ox_mass / ox_density) / (pi * tank_r^2);
        z_ox_fluid = (ox_tank_cg - ox_tank_h/2) + (h_ox_fluid / 2);
    else
        h_ox_fluid = 0; z_ox_fluid = 0;
    end

    %% 4. Calculate System Center of Gravity (CG)
    % Sum of Moments = sum(mass * position)
    moment_sum = ...
        engine_mass * engine_cg + ...
        fu_tank_mass * fu_tank_cg + ...
        ox_tank_mass * ox_tank_cg + ...
        structures_mass * structures_cg + ...
        avi_mass * avi_cg + ...
        fu_mass * z_fu_fluid + ...
        ox_mass * z_ox_fluid + ...
        m_ox_cap * z_ox_cap_bot + ... 
        m_ox_cap * z_ox_cap_top + ...  
        m_fu_cap * z_fu_cap_bot + ...  
        m_fu_cap * z_fu_cap_top;      

    total_mass = engine_mass + fu_tank_mass + ox_tank_mass + ...
                 structures_mass + avi_mass + fu_mass + ox_mass + ...
                 2 * m_ox_cap + 2 * m_fu_cap;

    if total_mass > 0
        cg = moment_sum / total_mass; % return 1
    else
        cg = 0;
    end

    %% 5. Calculate Moments of Inertia (MoI)
    % Anonymous functions for inertia - shout out gemini for this one
    calc_solid_Izz = @(m, r) 0.5 * m * r^2;
    calc_solid_Ixx = @(m, r, h) (1/12) * m * (3*r^2 + h^2);
    calc_hollow_Izz = @(m, ro, ri) 0.5 * m * (ro^2 + ri^2);
    calc_hollow_Ixx = @(m, ro, ri, h) (1/12) * m * (3*(ro^2 + ri^2) + h^2);

    % --- A. Engine ---
    Izz_eng = calc_solid_Izz(engine_mass, eng_r);
    Ixx_eng = calc_solid_Ixx(engine_mass, eng_r, eng_h) + engine_mass * (engine_cg - cg)^2;

    % --- B. Fuel Tank (Hollow Shell) ---
    r_in_fu = tank_r - fu_tank_wall_thick;
    Izz_fut = calc_hollow_Izz(fu_tank_mass, tank_r, r_in_fu);
    Ixx_fut = calc_hollow_Ixx(fu_tank_mass, tank_r, r_in_fu, fu_tank_h) + fu_tank_mass * (fu_tank_cg - cg)^2;

    % --- C. Oxidizer Tank (Hollow Shell) ---
    r_in_ox = tank_r - ox_tank_wall_thick;
    Izz_oxt = calc_hollow_Izz(ox_tank_mass, tank_r, r_in_ox);
    Ixx_oxt = calc_hollow_Ixx(ox_tank_mass, tank_r, r_in_ox, ox_tank_h) + ox_tank_mass * (ox_tank_cg - cg)^2;

    % --- D. Structures --- just asssume cylinder in it
    Izz_str = calc_solid_Izz(structures_mass, tank_r);
    Ixx_str = calc_solid_Ixx(structures_mass, tank_r, it_h) + structures_mass * (structures_cg - cg)^2;

    % --- E. Avionics --- just asssume cylinder in it
    Izz_avi = calc_solid_Izz(avi_mass, tank_r);
    Ixx_avi = calc_solid_Ixx(avi_mass, tank_r, it_h) + avi_mass * (avi_cg - cg)^2;

    % --- F. Fluids ---
    if fu_mass > 0
        Izz_fuf = calc_solid_Izz(fu_mass, tank_r);
        Ixx_fuf = calc_solid_Ixx(fu_mass, tank_r, h_fu_fluid) + fu_mass * (z_fu_fluid - cg)^2;
    else
        Izz_fuf = 0; Ixx_fuf = 0;
    end

    if ox_mass > 0
        Izz_oxf = calc_solid_Izz(ox_mass, tank_r);
        Ixx_oxf = calc_solid_Ixx(ox_mass, tank_r, h_ox_fluid) + ox_mass * (z_ox_fluid - cg)^2;
    else
        Izz_oxf = 0; Ixx_oxf = 0;
    end

    % --- G. End Caps ---
    % 1. Ox Caps (Solid Cylinders)
    % Izz is same for both
    Izz_ox_cap = calc_solid_Izz(m_ox_cap, tank_r);
    Ixx_ox_cap_local = calc_solid_Ixx(m_ox_cap, tank_r, h_ox_cap);
    
    Ixx_ox_caps_total = ...
        (Ixx_ox_cap_local + m_ox_cap * (z_ox_cap_bot - cg)^2) + ... % Bottom Cap
        (Ixx_ox_cap_local + m_ox_cap * (z_ox_cap_top - cg)^2);      % Top Cap

    % 2. Fuel Caps (Solid Cylinders)
    Izz_fu_cap = calc_solid_Izz(m_fu_cap, tank_r);
    Ixx_fu_cap_local = calc_solid_Ixx(m_fu_cap, tank_r, h_fu_cap);
    
    Ixx_fu_caps_total = ...
        (Ixx_fu_cap_local + m_fu_cap * (z_fu_cap_bot - cg)^2) + ... % Bottom Cap
        (Ixx_fu_cap_local + m_fu_cap * (z_fu_cap_top - cg)^2);      % Top Cap

    %% 6. Summation
    Izz_total = Izz_eng + Izz_fut + Izz_oxt + Izz_str + Izz_avi + ...
                Izz_fuf + Izz_oxf + ...
                2*Izz_ox_cap + 2*Izz_fu_cap;
                
    Ixx_total = Ixx_eng + Ixx_fut + Ixx_oxt + Ixx_str + Ixx_avi + ...
                Ixx_fuf + Ixx_oxf + ...
                Ixx_ox_caps_total + Ixx_fu_caps_total;
    
    Iyy_total = Ixx_total; % Symmetry

    MoI = [Ixx_total, 0, 0; 
           0, Iyy_total, 0; 
           0, 0, Izz_total]; % return 2
end
